simulink model "ClosedLoop_CqCsc"  (R2022b)
settings: Solver=VariableStepAuto  StartTime=0.0  StopTime=10.0  RelTol=1e-3
libraries: cstblocks x4
settings Model: Creator=antoninrenoir  LastModifiedBy=emili

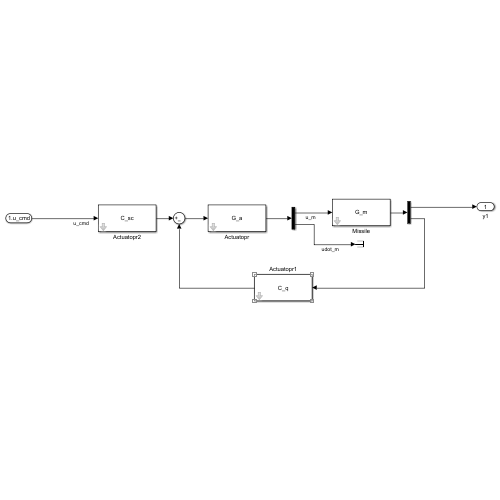
[thumbnail: Simulink's stored preview of the top-level diagram]
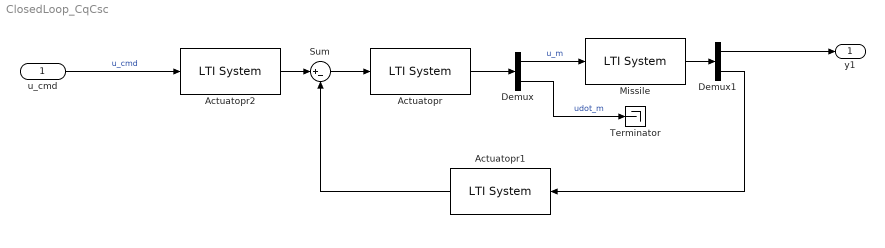
== system ClosedLoop_CqCsc ==
  u_cmd : Inport
  Actuatopr : cstblocks/LTI System  sys=G_a  IC=[]
  Actuatopr1 : cstblocks/LTI System  sys=C_q  IC=[]
  Actuatopr2 : cstblocks/LTI System  sys=C_sc  IC=[]
  Demux : Demux  Outputs=2
  Demux1 : Demux  Outputs=2
  Missile : cstblocks/LTI System  sys=G_m  IC=[]
  Sum : Sum  Inputs=|+-
  Terminator : Terminator
  y1 : Outport
  wires:
  Demux/1 -> Missile/1  "u_m"
  Missile/1 -> Demux1/1
  Actuatopr/1 -> Demux/1
  Demux/2 -> Terminator/1  "udot_m"
  u_cmd/1 -> Actuatopr2/1  "u_cmd"
  Demux1/1 -> y1/1
  Actuatopr2/1 -> Sum/1
  Sum/1 -> Actuatopr/1
  Actuatopr1/1 -> Sum/2
  Demux1/2 -> Actuatopr1/1
